simulink model "reference-tracking"  (R2025b)
settings: Solver=VariableStepAuto  StartTime=0.0  StopTime=600  RelTol=1e-3
libraries: fuzblock x1
settings Model: Creator=kicam  LastModifiedBy=kicam

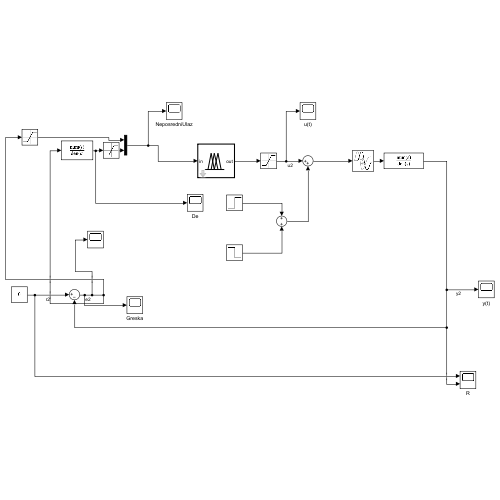
[thumbnail: Simulink's stored preview of the top-level diagram]
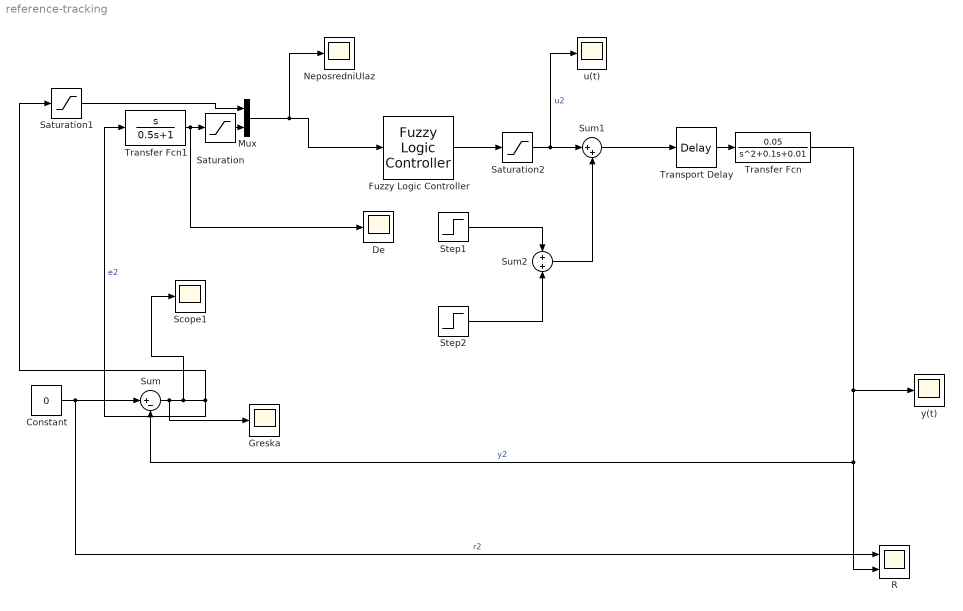
== system reference-tracking ==
  Constant : Constant  Value=0
  De : Scope
      settings: ActiveDisplayYMinimum=-1.7573178304996497  ActiveDisplayYMaximum=2.7359257839905569  DataLoggingVariableName=ScopeData5
  Fuzzy Logic Controller : fuzblock/Fuzzy Logic  Controller  FIS='mamdanitype1.fis'  OutputSampleNumber=101  DataType=double  UseLookupTable=off  NumBreakpoints=10  FuzzifiedInputs=off  RuleFiringStrengths=off  RuleOutputs=off  AggregatedOutputs=off  SimulateUsing=Interpreted execution  OutOfRangeInputValueMessage=warning  NoRuleFiredMessage=warning  EmptyOutputFuzzySetMessage=warning
  Greska : Scope
      settings: ActiveDisplayYMinimum=-23.066789148700124  ActiveDisplayYMaximum=26.621952024567872  DataLoggingVariableName=ScopeData4
  Mux : Mux  Inputs=2
  NeposredniUlaz : Scope
      settings: ActiveDisplayYMinimum=-23.066789148700124  ActiveDisplayYMaximum=26.621952024567872  DataLoggingVariableName=ScopeData6
  R : Scope  NumInputPorts=2
      settings: ActiveDisplayYMinimum=-21.425438753510917  ActiveDisplayYMaximum=60.123201686376063  DataLoggingVariableName=ScopeData3
  Saturation : Saturate  UpperLimit=20  LowerLimit=-20
  Saturation1 : Saturate  UpperLimit=50  LowerLimit=-50
  Saturation2 : Saturate  UpperLimit=10  LowerLimit=-10
  Scope1 : Scope
      settings: ActiveDisplayYMinimum=-1  ActiveDisplayYMaximum=1
  Step1 : Step  Time=10  After=5  SampleTime=0
  Step2 : Step  Time=150  After=-10  SampleTime=0
  Sum : Sum  Inputs=|+-
  Sum1 : Sum  Inputs=|++
  Sum2 : Sum
  Transfer Fcn : TransferFcn  Numerator=[0.05]  Denominator=[1 0.1 0.01]
  Transfer Fcn1 : TransferFcn  Numerator=[1 0]  Denominator=[0.5 1]
  Transport Delay : TransportDelay  DelayTime=2
  u(t) : Scope
      settings: ActiveDisplayYMinimum=-5.1682904519819255  ActiveDisplayYMaximum=6.1298100502202173  DataLoggingVariableName=ScopeData2
  y(t) : Scope
      settings: ActiveDisplayYMinimum=-1  ActiveDisplayYMaximum=1
  wires:
  Transfer Fcn1/1 -> De/1, Saturation/1
  Saturation/1 -> Mux/2
  Saturation1/1 -> Mux/1
  Transport Delay/1 -> Transfer Fcn/1
  Fuzzy Logic Controller/1 -> Saturation2/1
  Transfer Fcn/1 -> y(t)/1, Sum/2, R/2  "y2"
  Mux/1 -> NeposredniUlaz/1, Fuzzy Logic Controller/1
  Constant/1 -> R/1, Sum/1  "r2"
  Sum/1 -> Greska/1, Scope1/1, Saturation1/1, Transfer Fcn1/1  "e2"
  Saturation2/1 -> u(t)/1, Sum1/1  "u2"
  Sum1/1 -> Transport Delay/1
  Sum2/1 -> Sum1/2
  Step1/1 -> Sum2/1
  Step2/1 -> Sum2/2
